simulink model "collision"  (R2018a)
settings: Solver=FixedStepAuto  StartTime=0.0  StopTime=60  FixedStep=0.1  RelTol=1e-3
settings Model: Creator=besho  LastModifiedBy=besho

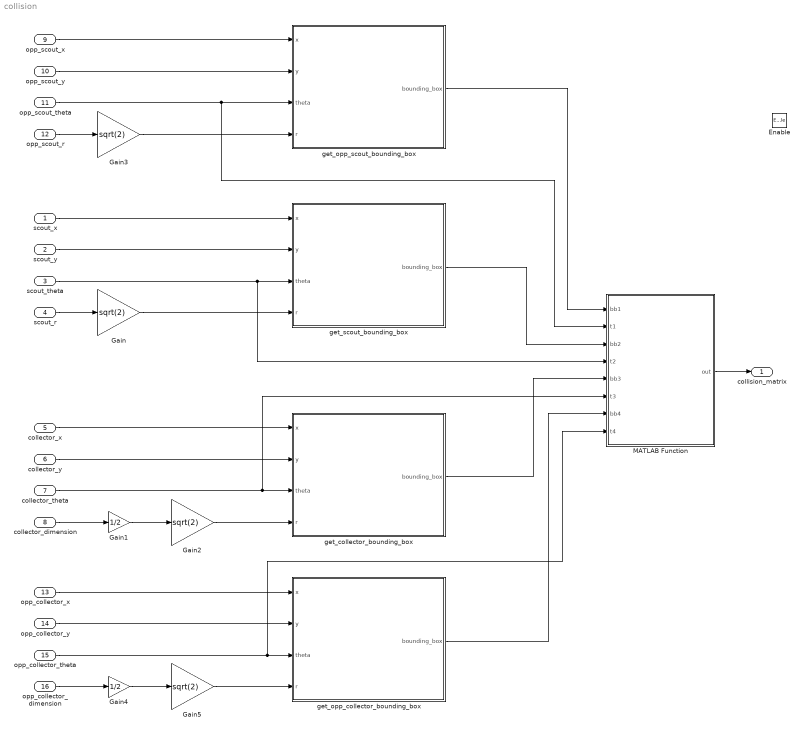
== system collision ==
  scout_x : Inport
  scout_y : Inport  Port=2
  scout_theta : Inport  Port=3
  scout_r : Inport  Port=4
  collector_x : Inport  Port=5
  collector_y : Inport  Port=6
  collector_theta : Inport  Port=7
  collector_dimension : Inport  Port=8
  opp_scout_x : Inport  Port=9
  opp_scout_y : Inport  Port=10
  opp_scout_theta : Inport  Port=11
  opp_scout_r : Inport  Port=12
  opp_collector_x : Inport  Port=13
  opp_collector_y : Inport  Port=14
  opp_collector_theta : Inport  Port=15
  opp_collector_dimension : Inport  Port=16
  Enable : EnablePort  StatesWhenEnabling=reset
  Gain{,2..3,5} (4 alike) : Gain  Gain=sqrt(2)
  Gain1 : Gain  Gain=1/2
  Gain4 : Gain  Gain=1/2
  MATLAB Function : MATLAB Function  TreatAsAtomicUnit=on
  get_collector_bounding_box : Subsystem  TreatAsAtomicUnit=on
  get_opp_collector_bounding_box : Subsystem  TreatAsAtomicUnit=on
  get_opp_scout_bounding_box : Subsystem  TreatAsAtomicUnit=on
  get_scout_bounding_box : Subsystem  TreatAsAtomicUnit=on
  collision_matrix : Outport
  wires:
  scout_r/1 -> Gain/1
  collector_dimension/1 -> Gain1/1
  Gain1/1 -> Gain2/1
  opp_scout_r/1 -> Gain3/1
  Gain4/1 -> Gain5/1
  opp_collector_dimension/1 -> Gain4/1
  Gain/1 -> get_scout_bounding_box/4(r)
  scout_theta/1 -> MATLAB Function/4(t2), get_scout_bounding_box/3(theta)
  scout_y/1 -> get_scout_bounding_box/2(y)
  scout_x/1 -> get_scout_bounding_box/1(x)
  Gain3/1 -> get_opp_scout_bounding_box/4(r)
  opp_scout_theta/1 -> MATLAB Function/2(t1), get_opp_scout_bounding_box/3(theta)
  opp_scout_y/1 -> get_opp_scout_bounding_box/2(y)
  opp_scout_x/1 -> get_opp_scout_bounding_box/1(x)
  collector_x/1 -> get_collector_bounding_box/1(x)
  collector_y/1 -> get_collector_bounding_box/2(y)
  collector_theta/1 -> MATLAB Function/6(t3), get_collector_bounding_box/3(theta)
  Gain2/1 -> get_collector_bounding_box/4(r)
  opp_collector_x/1 -> get_opp_collector_bounding_box/1(x)
  opp_collector_y/1 -> get_opp_collector_bounding_box/2(y)
  opp_collector_theta/1 -> MATLAB Function/8(t4), get_opp_collector_bounding_box/3(theta)
  Gain5/1 -> get_opp_collector_bounding_box/4(r)
  get_opp_scout_bounding_box/1(bounding_box) -> MATLAB Function/1(bb1)
  get_scout_bounding_box/1(bounding_box) -> MATLAB Function/3(bb2)
  get_collector_bounding_box/1(bounding_box) -> MATLAB Function/5(bb3)
  get_opp_collector_bounding_box/1(bounding_box) -> MATLAB Function/7(bb4)
  MATLAB Function/1(out) -> collision_matrix/1

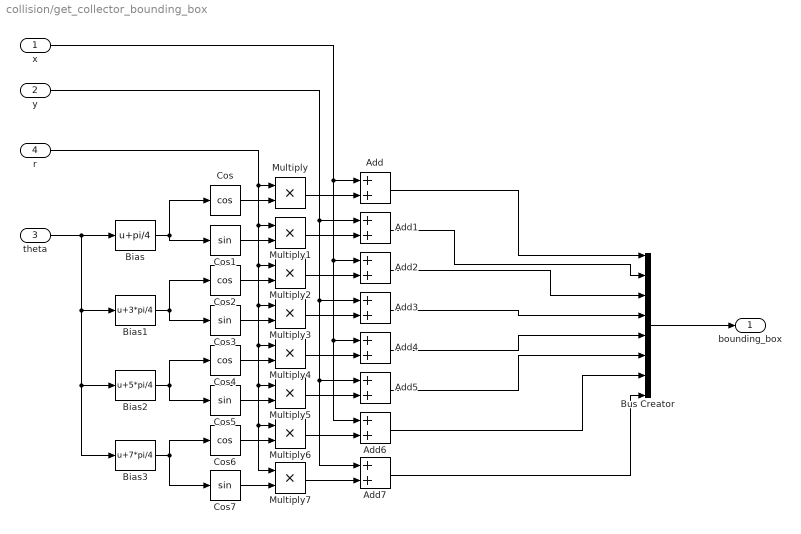
== system collision/get_collector_bounding_box ==
  x : Inport
  y : Inport  Port=2
  theta : Inport  Port=3
  r : Inport  Port=4
  Add{,1..7} (8 alike) : Sum
  Bias : Bias  Bias=pi/4
  Bias1 : Bias  Bias=3*pi/4
  Bias2 : Bias  Bias=5*pi/4
  Bias3 : Bias  Bias=7*pi/4
  Bus Creator : BusCreator  Inputs=8
  Cos{,2,4,6} (4 alike) : Trigonometry  Operator=cos
  Cos{1,3,5,7} (4 alike) : Trigonometry
  Multiply{,1..7} (8 alike) : Product
  bounding_box : Outport
  wires:
  Multiply5/1 -> Add5/2
  Multiply2/1 -> Add2/2
  Add1/1 -> Bus Creator/2
  Bias2/1 -> Cos5/1, Cos4/1
  Multiply4/1 -> Add4/2
  Add3/1 -> Bus Creator/4
  Cos3/1 -> Multiply3/2
  Add/1 -> Bus Creator/1
  Cos7/1 -> Multiply7/2
  Multiply3/1 -> Add3/2
  Bias1/1 -> Cos2/1, Cos3/1
  Cos2/1 -> Multiply2/2
  Bus Creator/1 -> bounding_box/1
  Cos4/1 -> Multiply4/2
  Cos5/1 -> Multiply5/2
  Bias3/1 -> Cos6/1, Cos7/1
  Add5/1 -> Bus Creator/6
  Cos/1 -> Multiply/2
  Multiply6/1 -> Add6/2
  Multiply7/1 -> Add7/2
  Add6/1 -> Bus Creator/7
  Multiply/1 -> Add/2
  Cos6/1 -> Multiply6/2
  Multiply1/1 -> Add1/2
  Bias/1 -> Cos/1, Cos1/1
  Add7/1 -> Bus Creator/8
  x/1 -> Add/1, Add2/1, Add4/1, Add6/1
  r/1 -> Multiply/1, Multiply1/1, Multiply2/1, Multiply3/1, Multiply4/1, Multiply5/1, Multiply6/1, Multiply7/1
  Cos1/1 -> Multiply1/2
  y/1 -> Add1/1, Add3/1, Add5/1, Add7/1
  theta/1 -> Bias/1, Bias1/1, Bias2/1, Bias3/1
  Add4/1 -> Bus Creator/5
  Add2/1 -> Bus Creator/3

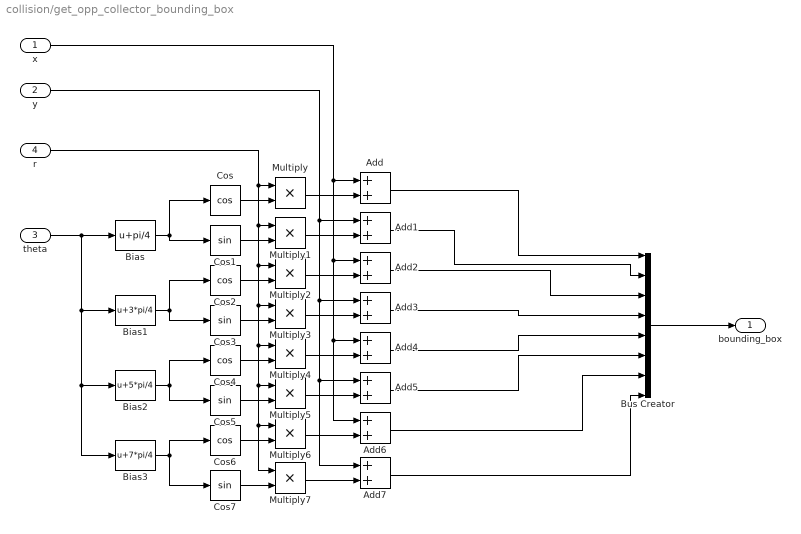
== system collision/get_opp_collector_bounding_box ==
  x : Inport
  y : Inport  Port=2
  theta : Inport  Port=3
  r : Inport  Port=4
  Add{,1..7} (8 alike) : Sum
  Bias : Bias  Bias=pi/4
  Bias1 : Bias  Bias=3*pi/4
  Bias2 : Bias  Bias=5*pi/4
  Bias3 : Bias  Bias=7*pi/4
  Bus Creator : BusCreator  Inputs=8
  Cos{,2,4,6} (4 alike) : Trigonometry  Operator=cos
  Cos{1,3,5,7} (4 alike) : Trigonometry
  Multiply{,1..7} (8 alike) : Product
  bounding_box : Outport
  wires:
  Multiply5/1 -> Add5/2
  Multiply2/1 -> Add2/2
  Add1/1 -> Bus Creator/2
  Bias2/1 -> Cos5/1, Cos4/1
  Multiply4/1 -> Add4/2
  Add3/1 -> Bus Creator/4
  Cos3/1 -> Multiply3/2
  Add/1 -> Bus Creator/1
  Cos7/1 -> Multiply7/2
  Multiply3/1 -> Add3/2
  Bias1/1 -> Cos2/1, Cos3/1
  Cos2/1 -> Multiply2/2
  Bus Creator/1 -> bounding_box/1
  Cos4/1 -> Multiply4/2
  Cos5/1 -> Multiply5/2
  Bias3/1 -> Cos6/1, Cos7/1
  Add5/1 -> Bus Creator/6
  Cos/1 -> Multiply/2
  Multiply6/1 -> Add6/2
  Multiply7/1 -> Add7/2
  Add6/1 -> Bus Creator/7
  Multiply/1 -> Add/2
  Cos6/1 -> Multiply6/2
  Multiply1/1 -> Add1/2
  Bias/1 -> Cos/1, Cos1/1
  Add7/1 -> Bus Creator/8
  x/1 -> Add/1, Add2/1, Add4/1, Add6/1
  r/1 -> Multiply/1, Multiply1/1, Multiply2/1, Multiply3/1, Multiply4/1, Multiply5/1, Multiply6/1, Multiply7/1
  Cos1/1 -> Multiply1/2
  y/1 -> Add1/1, Add3/1, Add5/1, Add7/1
  theta/1 -> Bias/1, Bias1/1, Bias2/1, Bias3/1
  Add4/1 -> Bus Creator/5
  Add2/1 -> Bus Creator/3

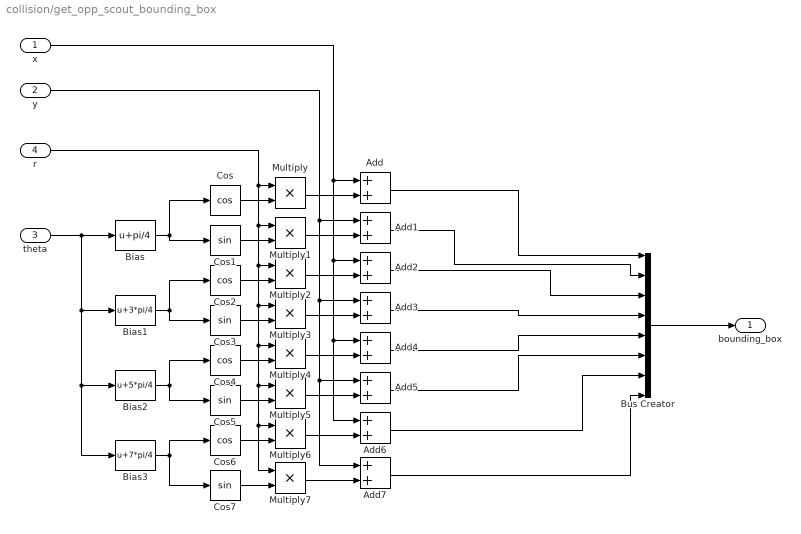
== system collision/get_opp_scout_bounding_box ==
  x : Inport
  y : Inport  Port=2
  theta : Inport  Port=3
  r : Inport  Port=4
  Add{,1..7} (8 alike) : Sum
  Bias : Bias  Bias=pi/4
  Bias1 : Bias  Bias=3*pi/4
  Bias2 : Bias  Bias=5*pi/4
  Bias3 : Bias  Bias=7*pi/4
  Bus Creator : BusCreator  Inputs=8
  Cos{,2,4,6} (4 alike) : Trigonometry  Operator=cos
  Cos{1,3,5,7} (4 alike) : Trigonometry
  Multiply{,1..7} (8 alike) : Product
  bounding_box : Outport
  wires:
  Multiply5/1 -> Add5/2
  Multiply2/1 -> Add2/2
  Add1/1 -> Bus Creator/2
  Bias2/1 -> Cos5/1, Cos4/1
  Multiply4/1 -> Add4/2
  Add3/1 -> Bus Creator/4
  Cos3/1 -> Multiply3/2
  Add/1 -> Bus Creator/1
  Cos7/1 -> Multiply7/2
  Multiply3/1 -> Add3/2
  Bias1/1 -> Cos2/1, Cos3/1
  Cos2/1 -> Multiply2/2
  Bus Creator/1 -> bounding_box/1
  Cos4/1 -> Multiply4/2
  Cos5/1 -> Multiply5/2
  Bias3/1 -> Cos6/1, Cos7/1
  Add5/1 -> Bus Creator/6
  Cos/1 -> Multiply/2
  Multiply6/1 -> Add6/2
  Multiply7/1 -> Add7/2
  Add6/1 -> Bus Creator/7
  Multiply/1 -> Add/2
  Cos6/1 -> Multiply6/2
  Multiply1/1 -> Add1/2
  Bias/1 -> Cos/1, Cos1/1
  Add7/1 -> Bus Creator/8
  x/1 -> Add/1, Add2/1, Add4/1, Add6/1
  r/1 -> Multiply/1, Multiply1/1, Multiply2/1, Multiply3/1, Multiply4/1, Multiply5/1, Multiply6/1, Multiply7/1
  Cos1/1 -> Multiply1/2
  y/1 -> Add1/1, Add3/1, Add5/1, Add7/1
  theta/1 -> Bias/1, Bias1/1, Bias2/1, Bias3/1
  Add4/1 -> Bus Creator/5
  Add2/1 -> Bus Creator/3

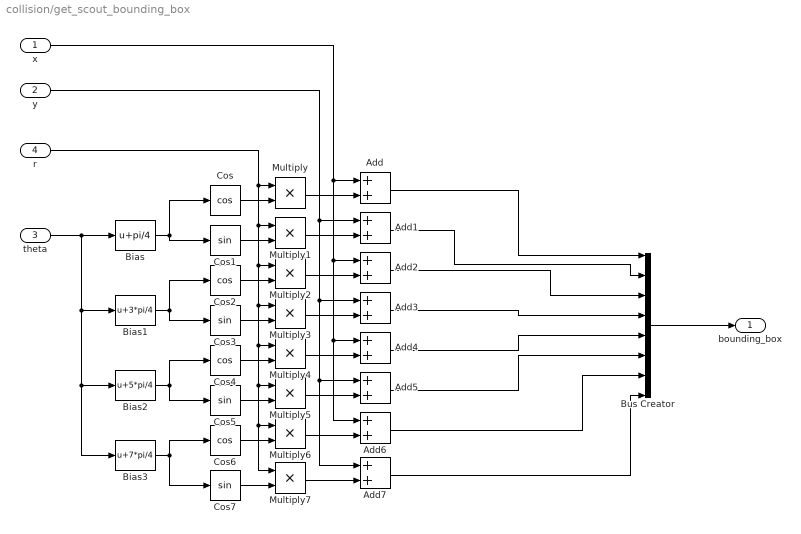
== system collision/get_scout_bounding_box ==
  x : Inport
  y : Inport  Port=2
  theta : Inport  Port=3
  r : Inport  Port=4
  Add{,1..7} (8 alike) : Sum
  Bias : Bias  Bias=pi/4
  Bias1 : Bias  Bias=3*pi/4
  Bias2 : Bias  Bias=5*pi/4
  Bias3 : Bias  Bias=7*pi/4
  Bus Creator : BusCreator  Inputs=8
  Cos{,2,4,6} (4 alike) : Trigonometry  Operator=cos
  Cos{1,3,5,7} (4 alike) : Trigonometry
  Multiply{,1..7} (8 alike) : Product
  bounding_box : Outport
  wires:
  Multiply5/1 -> Add5/2
  Multiply2/1 -> Add2/2
  Add1/1 -> Bus Creator/2
  Bias2/1 -> Cos5/1, Cos4/1
  Multiply4/1 -> Add4/2
  Add3/1 -> Bus Creator/4
  Cos3/1 -> Multiply3/2
  Add/1 -> Bus Creator/1
  Cos7/1 -> Multiply7/2
  Multiply3/1 -> Add3/2
  Bias1/1 -> Cos2/1, Cos3/1
  Cos2/1 -> Multiply2/2
  Bus Creator/1 -> bounding_box/1
  Cos4/1 -> Multiply4/2
  Cos5/1 -> Multiply5/2
  Bias3/1 -> Cos6/1, Cos7/1
  Add5/1 -> Bus Creator/6
  Cos/1 -> Multiply/2
  Multiply6/1 -> Add6/2
  Multiply7/1 -> Add7/2
  Add6/1 -> Bus Creator/7
  Multiply/1 -> Add/2
  Cos6/1 -> Multiply6/2
  Multiply1/1 -> Add1/2
  Bias/1 -> Cos/1, Cos1/1
  Add7/1 -> Bus Creator/8
  x/1 -> Add/1, Add2/1, Add4/1, Add6/1
  r/1 -> Multiply/1, Multiply1/1, Multiply2/1, Multiply3/1, Multiply4/1, Multiply5/1, Multiply6/1, Multiply7/1
  Cos1/1 -> Multiply1/2
  y/1 -> Add1/1, Add3/1, Add5/1, Add7/1
  theta/1 -> Bias/1, Bias1/1, Bias2/1, Bias3/1
  Add4/1 -> Bus Creator/5
  Add2/1 -> Bus Creator/3

== matlab function collision/MATLAB Function ==
  data: bb1 input; out output; t1 input; bb2 input; t2 input; bb3 input; t3 input; bb4 input; t4 input
function out = get_collisions(bb1, t1, bb2, t2, bb3, t3, bb4, t4)
coder.extrinsic('calc_collisions');
out = zeros(4,4);
out = calc_collisions([bb1, bb2, bb3, bb4], [t1, t2, t3, t4]);
end
